simulink model "ssc_aircraft_ecs_data"  (Simulink 9.1)
settings: Solver=VariableStepAuto  StartTime=0.0  StopTime=6000  RelTol=1e-3  AbsTol=1e-3
PreLoadFcn:
  | p_init = 101.325; % kPa
  | T_init = 45; % degC
  | RH_init = 0.5;
  | O3_init = 0.05e-6;
  | 
  | R_O3 = 173.218; % J/(kg*K)
  | 
  | flow_area = 0.016; % m^2
  | 
  | D_fuselage = 4; % m
  | L_fuselage = 35; % m
undefined symbols (not defined in the file or in its folder): sigbuilder_block
libraries: fl_lib x57, nesl_utility x24, simulink x6, HVAC_lib x4
(part 1 of 2)
Description:
  | Aircraft Environmental Control System
  | 
  | Copyright 2017-2018 The MathWorks, Inc.
CloseFcn:
  | try,close(h1_ssc_aircraft_ecs),end
  | clear h1_ssc_aircraft_ecs
  | try,close(h2_ssc_aircraft_ecs),end
  | clear h2_ssc_aircraft_ecs
  | try,close(h3_ssc_aircraft_ecs),end
  | clear h3_ssc_aircraft_ecs
  | try,close(h4_ssc_aircraft_ecs),end
  | clear h4_ssc_aircraft_ecs
  | 
  | clear tout simlog_ssc_aircraft_ecs
  | clear p_init T_init RH_init O3_init R_O3 flow_area D_fuselage L_fuselage
settings Model: Creator=MathWorks  LastModifiedBy=ZENLAB-328
settings SolverCC: MaxConsecutiveMinStep=2
settings DataIOCC: SaveFormat=Dataset
settings OptimizationCC: LifeSpan=auto
settings DebuggingCC: UnderspecifiedInitializationDetection=Simplified  MergeDetectMultiDrivingBlocksExec=error  SFUnexpectedBacktrackingDiag=error  SFNoUnconditionalDefaultTransitionDiag=error  SFExecutionAtInitializationDiag=warning
settings HardwareCC: ProdBitPerPointer=64  ProdBitPerSizeT=64  ProdBitPerPtrDiffT=64  ProdLargestAtomicFloat=Float  ProdIntDivRoundTo=Zero  ProdEndianess=LittleEndian  ProdWordSize=64  ProdHWDeviceType=Intel->x86-64 (Windows64)
settings ModelReferenceCC: PropagateSignalLabelsOutOfModel=on
settings CodeAppCC: StateflowObjectComments=off
settings GRTTargetCC: TargetLangStandard=C99 (ISO)  CombineOutputUpdateFcns=on  GRTInterface=off
settings ConfigComp: CovMetricSettings=dwe  CovHtmlReporting=off  CovSaveCumulativeToWorkspaceVar=off  CovSaveSingleToWorkspaceVar=off  CovExternalEMLEnable=on
settings SimscapeCC: SimscapeLogType=all  SimscapeLogSimulationStatistics=on  SimscapeLogName=simlog_ssc_aircraft_ecs  SimscapeLogDataHistory=10000

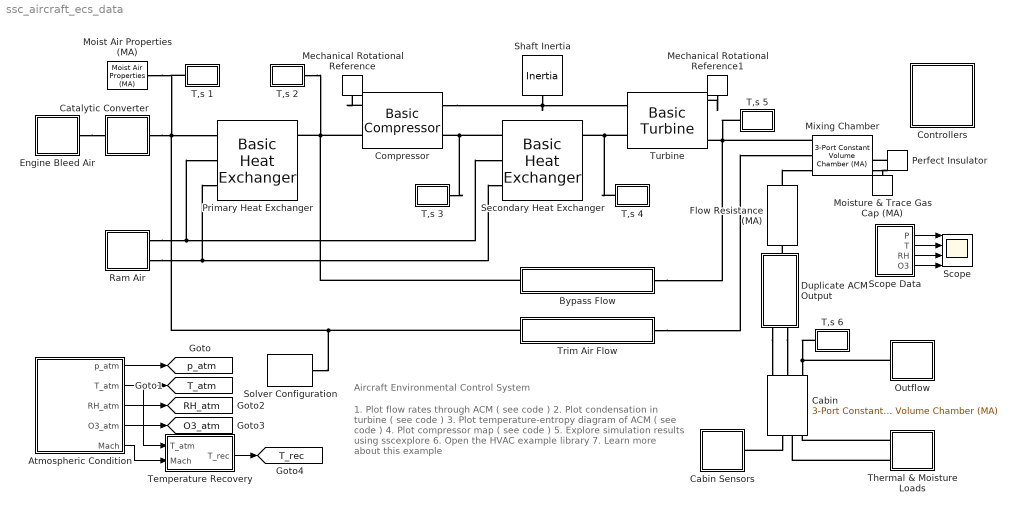
== system ssc_aircraft_ecs_data ==
  note: Aircraft Environmental Control System
  note: 1. Plot flow rates through ACM ( see code )
      | 2. Plot condensation in turbine ( see code )
      | 3. Plot temperature-entropy diagram of ACM ( see code )
      | 4. Plot compressor map ( see code )
      | 5. Explore simulation results using sscexplore
      | 6. Open the HVAC example library
      | 7. Learn more about this example
  Atmospheric Condition : Subsystem  Tag=STV Subsys  LoadFcn=sigbuilder_block('load');  StartFcn=sigbuilder_block('start');  StopFcn=sigbuilder_block('stop');  ClipboardFcn=sigbuilder_block('clipboard');  mask(Sigbuilder block){tuvar=[0:10]}
      mask help: Simulink:masks:SigbuilderBlock_MD
      mask init:
      | if ~strcmp(get_param(bdroot(gcbh),'SimulationStatus'),'stopped') tuvar = sigbuilder_block('maskInit'); end
      settings: CopyFcn=sigbuilder_block('copy');  DeleteFcn=sigbuilder_block('delete');  ModelCloseFcn=sigbuilder_block('modelClose');  PreSaveFcn=sigbuilder_block('preSave');  PauseFcn=sigbuilder_block('pause');  ContinueFcn=sigbuilder_block('continue');  NameChangeFcn=sigbuilder_block('namechange');  OpenFcn=sigbuilder_block('open',[42.75 9 1391.25 641.25 ]);  CloseFcn=sigbuilder_block('close');
      mask Display: plot(0, 0, 100, 100,[2, 2, 32, 32, 2], [68, 8, 8, 68, 68],[32, 2], [38, 38], [32, 19, 2],[53, 60, 44], [32, 17, 17, 2],[16, 16, 31, 31]);txt = getActiveGroup(gcbh);text(2, 100, txt,'verticalAlignment', 'top');
  Bypass Flow : Subsystem  Tag=PublishSubsystem
  Cabin : fl_lib/Moist Air/Elements/3-Port Constant Volume Chamber (MA)  volume=pi*D_fuselage^2/4 * L_fuselage m^3  area_A=flow_area m^2  area_B=flow_area m^2  area_C=flow_area m^2  RH_ws=1  time_constant=1e-3 s  p_I_specify=on  p_I_priority=High  p_I=p_init kPa  p_I_nominal_specify=off  p_I_nominal_unit=MPa  p_I_nominal_value=1  T_I_specify=on  T_I_priority=High  T_I=T_init degC  T_I_nominal_specify=off  T_I_nominal_unit=K  T_I_nominal_value=1  RH_I_specify=on  RH_I_priority=High  RH_I=RH_init  RH_I_nominal_specify=off  RH_I_nominal_unit=1  RH_I_nominal_value=1  x_w_I_specify=off  x_w_I_priority=None  x_w_I=0  x_w_I_nominal_specify=off  x_w_I_nominal_unit=1  x_w_I_nominal_value=1  y_w_I_specify=off  y_w_I_priority=None  y_w_I=0  y_w_I_nominal_specify=off  y_w_I_nominal_unit=1  y_w_I_nominal_value=1  HR_I_specify=off  HR_I_priority=None  HR_I=0  HR_I_nominal_specify=off  HR_I_nominal_unit=1  HR_I_nominal_value=1  x_g_I_specify=on  x_g_I_priority=None  x_g_I=0  x_g_I_nominal_specify=off  x_g_I_nominal_unit=1  x_g_I_nominal_value=1  y_g_I_specify=on  y_g_I_priority=High  y_g_I=O3_init  y_g_I_nominal_specify=off  y_g_I_nominal_unit=1  y_g_I_nominal_value=1  t_specify=off  t_priority=High  t=0 s  t_nominal_specify=off  t_nominal_unit=s  t_nominal_value=1
      settings: SourceProductName=Simscape  SourceProductBaseCode=SS
  Cabin Sensors : Subsystem
  Catalytic Converter : Subsystem  Tag=PublishSubsystem  mask(Catalytic Converter){}
      mask help: This subsystem removes ozone (O3) from the air flow at the specified removal rate.
      mask init:
      | removal_rate=evalin('base','Foz')
  Compressor : HVAC_lib/Basic Compressor  pr_des=2  mdot_corr_des=0.5 kg/s  omega_corr_des=4e4 rpm  p_ref=0.101325 MPa  T_ref=288.15 K  RH_ref=0  b1=1.5  b2=0.7  b3=0.08  eta_poly=0.92  eta_mech=0.98  area_A=flow_area m^2  area_B=flow_area/2 m^2  mdot_A_specify=off  mdot_A_priority=None  mdot_A=0 kg/s  mdot_A_nominal_specify=off  mdot_A_nominal_unit=kg/s  mdot_A_nominal_value=1  mdot_B_specify=off  mdot_B_priority=None  mdot_B=0 kg/s  mdot_B_nominal_specify=off  mdot_B_nominal_unit=kg/s  mdot_B_nominal_value=1  Phi_A_specify=off  Phi_A_priority=None  Phi_A=0 kW  Phi_A_nominal_specify=off  Phi_A_nominal_unit=kW  Phi_A_nominal_value=1  Phi_B_specify=off  Phi_B_priority=None  Phi_B=0 kW  Phi_B_nominal_specify=off  Phi_B_nominal_unit=kW  Phi_B_nominal_value=1  mdot_w_A_specify=off  mdot_w_A_priority=None  mdot_w_A=0 kg/s  mdot_w_A_nominal_specify=off  mdot_w_A_nominal_unit=kg/s  mdot_w_A_nominal_value=1  mdot_w_B_specify=off  mdot_w_B_priority=None  mdot_w_B=0 kg/s  mdot_w_B_nominal_specify=off  mdot_w_B_nominal_unit=kg/s  mdot_w_B_nominal_value=1  mdot_g_A_specify=off  mdot_g_A_priority=None  mdot_g_A=0 kg/s  mdot_g_A_nominal_specify=off  mdot_g_A_nominal_unit=kg/s  mdot_g_A_nominal_value=1  mdot_g_B_specify=off  mdot_g_B_priority=None  mdot_g_B=0 kg/s  mdot_g_B_nominal_specify=off  mdot_g_B_nominal_unit=kg/s  mdot_g_B_nominal_value=1  torque_specify=off  torque_priority=None  torque=1 N*m  torque_nominal_specify=off  torque_nominal_unit=N*m  torque_nominal_value=1  mechanical_power_specify=off  mechanical_power_priority=None  mechanical_power=1 kW  mechanical_power_nominal_specify=off  mechanical_power_nominal_unit=kW  mechanical_power_nominal_value=1  fluid_power_specify=off  fluid_power_priority=None  fluid_power=1 kW  fluid_power_nominal_specify=off  fluid_power_nominal_unit=kW  fluid_power_nominal_value=1  T_in_specify=off  T_in_priority=None  T_in=300 K  T_in_nominal_specify=off  T_in_nominal_unit=K  T_in_nominal_value=1  T_out_specify=off  T_out_priority=None  T_out=300 K  T_out_nominal_specify=off  T_out_nominal_unit=K  T_out_nominal_value=1
  Controllers : Subsystem  Tag=PublishSubsystem  mask(Controllers){T_turbine_setpoint=0, T_cabin_setpoint=22, p_cabin_min=80}
      mask prompts: T_turbine_setpoint "Turbine outlet temperature (degC)"; T_cabin_setpoint "Cabin temperature (degC)"; p_cabin_min "Minimum cabin pressure (kPa)"
      mask help: This subsystem contains the 4 controllers that regulate the flow in the air cycle machine (ACM) to achieve the following desired conditions.
      mask init:
      | mdot_setpoint=evalin('base','flowrate')
  Duplicate ACM Output : Subsystem  mask(Duplicate ACM Output){}
      mask help: This subsystem provides a second stream of conditioned air flow that mirrors the output of the first air cycle machine (ACM) without actually modeling the second ACM.
  Engine Bleed Air : Subsystem  Tag=PublishSubsystem  mask(Engine Bleed Air){p_bleed=250, T_bleed=180}
      mask prompts: p_bleed "Bleed air pressure (kPa)"; T_bleed "Bleed air temperature (degC)"
      mask help: This subsystem models the supply of hot, pressurized air to the air cycle machine (ACM) at a controlled flow rate.
  Flow Resistance (MA) : fl_lib/Moist Air/Elements/Flow Resistance (MA)  delta_p_nominal=1 kPa  mdot_nominal=1 kg/s  rho_nominal=1.2 kg/m^3  area=flow_area m^2  laminar_fraction=1e-3
      settings: SourceProductName=Simscape  SourceProductBaseCode=SS
  Mechanical Rotational Reference : fl_lib/Mechanical/Rotational Elements/Mechanical Rotational Reference
  Mechanical Rotational Reference1 : fl_lib/Mechanical/Rotational Elements/Mechanical Rotational Reference
  Mixing Chamber : fl_lib/Moist Air/Elements/3-Port Constant Volume Chamber (MA)  volume=0.001 m^3  area_A=flow_area m^2  area_B=flow_area m^2  area_C=flow_area m^2  RH_ws=1  time_constant=1e-3 s  p_I_specify=on  p_I_priority=High  p_I=p_init kPa  p_I_nominal_specify=off  p_I_nominal_unit=MPa  p_I_nominal_value=1  T_I_specify=on  T_I_priority=High  T_I=T_init degC  T_I_nominal_specify=off  T_I_nominal_unit=K  T_I_nominal_value=1  RH_I_specify=on  RH_I_priority=High  RH_I=RH_init  RH_I_nominal_specify=off  RH_I_nominal_unit=1  RH_I_nominal_value=1  x_w_I_specify=off  x_w_I_priority=None  x_w_I=0  x_w_I_nominal_specify=off  x_w_I_nominal_unit=1  x_w_I_nominal_value=1  y_w_I_specify=off  y_w_I_priority=None  y_w_I=0  y_w_I_nominal_specify=off  y_w_I_nominal_unit=1  y_w_I_nominal_value=1  HR_I_specify=off  HR_I_priority=None  HR_I=0  HR_I_nominal_specify=off  HR_I_nominal_unit=1  HR_I_nominal_value=1  x_g_I_specify=on  x_g_I_priority=None  x_g_I=0  x_g_I_nominal_specify=off  x_g_I_nominal_unit=1  x_g_I_nominal_value=1  y_g_I_specify=on  y_g_I_priority=High  y_g_I=O3_init  y_g_I_nominal_specify=off  y_g_I_nominal_unit=1  y_g_I_nominal_value=1  t_specify=off  t_priority=High  t=0 s  t_nominal_specify=off  t_nominal_unit=s  t_nominal_value=1
      settings: SourceProductName=Simscape  SourceProductBaseCode=SS
  Moist Air Properties (MA) : fl_lib/Moist Air/Utilities/Moist Air Properties (MA)  trace_gas_model=2  R_a=287.047 J/kg/K  R_w=461.523 J/kg/K  R_g=R_O3 J/kg/K  T_TLU=[-56.55, -50 : 10 : -10, -5 : 1 : 5, 10 : 10 : 350]' degC  p_ws_TLU=[1.71168953425982e-06; 3.93770601979424e-06; 1.28411717710344e-05; 3.80051394873809e-05; .00010323902900209; .000259873810798063; .000401741022116384; .000437454836117844; .000476040820618202; .000517704666185737; .000562664883741207; .000611212677444345; .000657088049117899; .000705987905898279; .000758082381149132; .000813549384183233; .000872574861129522; .00122818386934022; .0023392147667769; .00424668834054807; .00738442748706953; .0123512704340234; .0199458019246787; .0312006356960619; .0474147199263783; .0701823607447713; .10141797792131; .143375967241115; .198665399739302; .270259606559999; .361500961984849; .476101381081492; .618139196722055; .792053183687694; 1.0026345688121; 1.25501792086105; 1.55467186826983; 1.90739066433297; 2.31928772772542; 2.79679245576864; 3.34665187151016; 3.97593907083533; 4.69207105435535; 5.5028394740883; 6.41645928168037; 7.4416425436169; 8.58770832955728; 9.86474556030261; 11.2838558865497; 12.8575218898034; 14.6001810568052; 16.5291642526045] MPa  h_w_vap_TLU=[2836.88241275372; 2837.81392500514; 2838.63937175807; 2838.7309929628; 2838.06905313927; 2836.62597341095; 2835.60023952573; 2835.37006381376; 2835.13143158077; 2834.88429145066; 2834.62859062897; 2500.93420564316; 2498.55329907119; 2496.17495082036; 2493.79885912205; 2491.42474723191; 2489.05236104642; 2477.20875029194; 2453.54955988604; 2429.83856603313; 2406.00136954922; 2381.97406342174; 2357.69101156389; 2333.08088387814; 2308.06565480412; 2282.56034405021; 2256.47287422313; 2229.70428017508; 2202.14968030993; 2173.69998896199; 2144.24368406447; 2113.66758247452; 2081.85585110571; 2048.68725710494; 2014.03141249899; 1977.7449923284; 1939.66849592886; 1899.62342931686; 1857.40930169838; 1812.79975416601; 1765.53721731251; 1715.32525772152; 1661.81700477787; 1604.59703745016; 1543.1534616334; 1476.83692476464; 1404.80240352424; 1325.92091736114; 1238.61667822208; 1140.5102987018; 1027.62017777647; 892.733785613825] kJ/kg  h_a_TLU=[342.416126230579; 349.005511058471; 359.063577249119; 369.119948684177; 379.175469465129; 389.230944678417; 394.258910928084; 395.264534937366; 396.27017101329; 397.275819932805; 398.281482472874; 399.287159410541; 400.292851523015; 401.298559587728; 402.304284382408; 403.310026685143; 404.315787274435; 409.34489180313; 419.404921755863; 429.468036401264; 439.535033154839; 449.606720928652; 459.683919949603; 469.767460521911; 479.858181001348; 489.956925196484; 500.064539372946; 510.181869006204; 520.309755403634; 530.449032296018; 540.60052248087; 550.765034584465; 560.943359995745; 571.136270013102; 581.344513234296; 591.568813210327; 601.809866375885; 612.068340261954; 622.344871990218; 632.640067043998; 642.95449830646; 653.288705353699; 663.643193987949; 674.018435994423; 684.414869104228; 694.832897145098; 705.272890361557; 715.735185886199; 726.220088344236; 736.727870574087; 747.258774447567; 757.813011774199] kJ/kg  h_w_TLU=[2396.55944251649; 2408.68643343608; 2427.1988031141; 2445.702165897; 2464.18429108356; 2482.62529466839; 2491.82135326629; 2493.6580151792; 2495.49372578218; 2497.32843835745; 2499.16210446923; 2500.99462758899; 2502.83092214066; 2504.6665223621; 2506.50140563013; 2508.335548891; 2510.16892865793; 2519.32352241995; 2537.56068088674; 2555.67742615292; 2573.6403223998; 2591.4109179101; 2608.9455037701; 2626.19492016262; 2643.10444358428; 2659.61377634497; 2675.58278696023; 2696.1846256545; 2716.49989553741; 2736.6235210957; 2756.61216047011; 2776.50561773853; 2796.33378922508; 2816.11979583049; 2835.88181423877; 2855.63430574511; 2875.38889327595; 2895.15500577172; 2914.94035964689; 2934.75132290228; 2954.59319330244; 2974.47041285505; 2994.38673458964; 3014.34535328009; 3034.34900867103; 3054.40006755764; 3074.50058946898; 3094.65237953784; 3114.85703128106; 3135.11596137801; 3155.43043805905; 3175.80160435813] kJ/kg  h_g_TLU=-1 kJ/kg  mu_a_TLU=[14.2568883320012; 14.6140127728333; 15.1517277055779; 15.6806860159119; 16.2012351072083; 16.7137043125028; 16.9670071730589; 17.017438062815; 17.0677930842452; 17.1180725309876; 17.1682766951315; 17.2184058672268; 17.2684603362935; 17.3184403898301; 17.3683463138234; 17.4181783927569; 17.4679369096204; 17.7156358640698; 18.2056751785154; 18.68879035749; 19.1652344664982; 19.6352478927873; 20.099059103658; 20.5568853601578; 21.0089333871663; 21.4554000014051; 21.8964726992323; 22.3323302062775; 22.7631429910631; 23.1890737447833; 23.6102778293792; 24.0269036959922; 24.4390932757886; 24.8469823450548; 25.2507008663546; 25.6503733074314; 26.0461189394339; 26.4380521159325; 26.8262825340948; 27.2109154792923; 27.5920520543128; 27.969789394274; 28.3442208682439; 28.7154362685068; 29.0835219883356; 29.4485611890712; 29.8106339572472; 30.1698174524429; 30.5261860464955; 30.8798114546565; 31.2307628592324; 31.5791070262086] s*uPa  mu_w_TLU=[6.81365662228272; 7.04953750742707; 7.40970098298307; 7.76991278093907; 8.13017290129507; 8.49048134405107; 8.67065368632907; 8.70668960445667; 8.74272600580827; 8.77876289038387; 8.81480025818347; 8.85083810920707; 8.88687644345467; 8.92291526092627; 8.95895456162187; 8.99499434554147; 9.03103461268507; 9.21124319676307; 9.57169660671907; 9.93219833907507; 10.2927483938311; 10.6533467709871; 11.0139934705431; 11.3746884924991; 11.7354318368551; 12.0962235036111; 12.4570634927671; 12.8179518043231; 13.1788884382791; 13.5398733946351; 13.9009066733911; 14.2619882745471; 14.6231181981031; 14.9842964440591; 15.3455230124151; 15.7067979031711; 16.0681211163271; 16.4294926518831; 16.7909125098391; 17.1523806901951; 17.5138971929511; 17.8754620181071; 18.2370751656631; 18.5987366356191; 18.9604464279751; 19.3222045427311; 19.6840109798871; 20.0458657394431; 20.4077688213991; 20.7697202257551; 21.1317199525111; 21.4937680016671] s*uPa  mu_g_TLU=-1 s*uPa  k_a_TLU=[19.8808489374933; 20.4162454629695; 21.2248743590758; 22.0232452890903; 22.8117314495857; 23.5906913619588; 23.9767075412237; 24.053639990175; 24.1304826682191; 24.2072359051629; 24.2839000294007; 24.3604753679152; 24.4369622462801; 24.5133609886625; 24.5896719178249; 24.6658953551279; 24.7420316205333; 25.1214164701832; 25.8738283029331; 26.6180150229276; 27.3542674377332; 28.0828634735341; 28.8040686837224; 29.5181367785657; 30.2253101618423; 30.9258204644224; 31.6198890677835; 32.3077276126633; 32.9895384896798; 33.6655153099498; 34.33584335461; 35.0007000027879; 35.6602551380254; 36.3146715334901; 36.9641052165342; 37.6087058133173; 38.248616874307; 38.8839761815308; 39.5149160384798; 40.1415635435708; 40.7640408480637; 41.3824653993118; 41.9969501701893; 42.6076038755117; 43.2145311762238; 43.8178328720941; 44.4176060836121; 45.013944423749; 45.6069381602018; 46.1966743687041; 46.783237077953; 47.3667074066625] mW/m/K  k_w_TLU=[11.46288215976; 11.941997488935; 12.676358586935; 13.414208884935; 14.155548382935; 14.900377080935; 15.274099879935; 15.348949115735; 15.423833243535; 15.498752263335; 15.573706175135; 15.648694978935; 15.723718674735; 15.798777262535; 15.873870742335; 15.948999114135; 16.024162377935; 16.400502076935; 17.155798374935; 17.914583872935; 18.676858570935; 19.442622468935; 20.211875566935; 20.984617864935; 21.760849362935; 22.540570060935; 23.323779958935; 24.110479056935; 24.900667354935; 25.694344852935; 26.491511550935; 27.292167448935; 28.096312546935; 28.903946844935; 29.715070342935; 30.529683040935; 31.347784938935; 32.169376036935; 32.994456334935; 33.823025832935; 34.655084530935; 35.490632428935; 36.329669526935; 37.172195824935; 38.018211322935; 38.867716020935; 39.720709918935; 40.577193016935; 41.437165314935; 42.300626812935; 43.167577510935; 44.038017408935] mW/m/K  k_g_TLU=-1 mW/m/K  D_w=25 mm^2/s  D_g=16 mm^2/s  p_min=1 kPa  p_max=inf MPa  T_min=-56.55 degC  T_max=350 degC  p_atm=0.101325 MPa  T_atm=20 degC
      settings: SourceProductName=Simscape  SourceProductBaseCode=SS
  Moisture & Trace Gas Cap (MA) : fl_lib/Moist Air/Sources/Moisture & Trace Gas Sources/Moisture & Trace Gas Cap (MA)
      settings: SourceProductName=Simscape  SourceProductBaseCode=SS
  Outflow : Subsystem  Tag=PublishSubsystem
  Perfect Insulator : fl_lib/Thermal/Thermal Elements/Perfect Insulator  T_specify=off  T_priority=None  T=0 K  T_nominal_specify=off  T_nominal_unit=K  T_nominal_value=1
      settings: SourceProductName=Simscape
  Primary Heat Exchanger : HVAC_lib/Basic Heat Exchanger  Q_des=100 kW  T1_des=180 degC  mdot1_des=1 kg/s  cp1_des=1.02 kJ/kg/K  Dp1_des=20 kPa  T2_des=45 degC  mdot2_des=3 kg/s  cp2_des=1.007 kJ/kg/K  volume=0.025 m^3  port_area=flow_area m^2  RH_ws=1  time_constant=1e-3 s  p_I_specify=on  p_I_priority=High  p_I=p_init kPa  p_I_nominal_specify=off  p_I_nominal_unit=MPa  p_I_nominal_value=1  T_I_specify=on  T_I_priority=High  T_I=T_init degC  T_I_nominal_specify=off  T_I_nominal_unit=K  T_I_nominal_value=1  RH_I_specify=on  RH_I_priority=High  RH_I=RH_init  RH_I_nominal_specify=off  RH_I_nominal_unit=1  RH_I_nominal_value=1  x_w_I_specify=off  x_w_I_priority=None  x_w_I=0  x_w_I_nominal_specify=off  x_w_I_nominal_unit=1  x_w_I_nominal_value=1  y_w_I_specify=off  y_w_I_priority=None  y_w_I=0  y_w_I_nominal_specify=off  y_w_I_nominal_unit=1  y_w_I_nominal_value=1  HR_I_specify=off  HR_I_priority=None  HR_I=0  HR_I_nominal_specify=off  HR_I_nominal_unit=1  HR_I_nominal_value=1  x_g_I_specify=on  x_g_I_priority=None  x_g_I=0  x_g_I_nominal_specify=off  x_g_I_nominal_unit=1  x_g_I_nominal_value=1  y_g_I_specify=on  y_g_I_priority=High  y_g_I=O3_init  y_g_I_nominal_specify=off  y_g_I_nominal_unit=1  y_g_I_nominal_value=1  mdot_A_specify=off  mdot_A_priority=None  mdot_A=0 kg/s  mdot_A_nominal_specify=off  mdot_A_nominal_unit=kg/s  mdot_A_nominal_value=1  mdot_B_specify=off  mdot_B_priority=None  mdot_B=0 kg/s  mdot_B_nominal_specify=off  mdot_B_nominal_unit=kg/s  mdot_B_nominal_value=1  Phi_A_specify=off  Phi_A_priority=None  Phi_A=0 kW  Phi_A_nominal_specify=off  Phi_A_nominal_unit=kW  Phi_A_nominal_value=1  Phi_B_specify=off  Phi_B_priority=None  Phi_B=0 kW  Phi_B_nominal_specify=off  Phi_B_nominal_unit=kW  Phi_B_nominal_value=1  mdot_w_A_specify=off  mdot_w_A_priority=None  mdot_w_A=0 kg/s  mdot_w_A_nominal_specify=off  mdot_w_A_nominal_unit=kg/s  mdot_w_A_nominal_value=1  mdot_w_B_specify=off  mdot_w_B_priority=None  mdot_w_B=0 kg/s  mdot_w_B_nominal_specify=off  mdot_w_B_nominal_unit=kg/s  mdot_w_B_nominal_value=1  mdot_g_A_specify=off  mdot_g_A_priority=None  mdot_g_A=0 kg/s  mdot_g_A_nominal_specify=off  mdot_g_A_nominal_unit=kg/s  mdot_g_A_nominal_value=1  mdot_g_B_specify=off  mdot_g_B_priority=None  mdot_g_B=0 kg/s  mdot_g_B_nominal_specify=off  mdot_g_B_nominal_unit=kg/s  mdot_g_B_nominal_value=1  rho_I_specify=off  rho_I_priority=None  rho_I=1.2 kg/m^3  rho_I_nominal_specify=off  rho_I_nominal_unit=kg/m^3  rho_I_nominal_value=1  h_I_specify=off  h_I_priority=None  h_I=420 kJ/kg  h_I_nominal_specify=off  h_I_nominal_unit=kJ/kg  h_I_nominal_value=1  x_a_I_specify=off  x_a_I_priority=None  x_a_I=1  x_a_I_nominal_specify=off  x_a_I_nominal_unit=1  x_a_I_nominal_value=1  effectiveness_specify=off  effectiveness_priority=None  effectiveness=1  effectiveness_nominal_specify=off  effectiveness_nominal_unit=1  effectiveness_nominal_value=1  Q_hex_specify=off  Q_hex_priority=None  Q_hex=0 kW  Q_hex_nominal_specify=off  Q_hex_nominal_unit=kW  Q_hex_nominal_value=1  p_ws_ratio_I_specify=off  p_ws_ratio_I_priority=None  p_ws_ratio_I=1  p_ws_ratio_I_nominal_specify=off  p_ws_ratio_I_nominal_unit=1  p_ws_ratio_I_nominal_value=1  t_specify=off  t_priority=High  t=0 s  t_nominal_specify=off  t_nominal_unit=s  t_nominal_value=1
  Ram Air : Subsystem  mask(Ram Air){mdot_ram=3}
      mask prompts: mdot_ram "Ram air mass flow rate (kg/s)"
      mask help: This subsystem represents the air from the external environment that is used as the coolant for the heat exchangers in the air cycle machine (ACM).
  Scope : Scope  NumInputPorts=4
  Scope Data : Subsystem
      mask init:
      | %set_param([gcb,'/To Workspace'], 'VariableName', p_atm);
      | %set_param([gcb,'/To Workspace'], 'VariableName', p_cabin);
      | %set_param([gcb,'/To Workspace'], 'VariableName', T_cabin);
      | %set_param([gcb,'/To Workspace'], 'VariableName', RH_cabin);
      | %set_param([gcb,'/To Workspace'], 'VariableName', Q3_cabin);
  Secondary Heat Exchanger : HVAC_lib/Basic Heat Exchanger  Q_des=150 kW  T1_des=180 degC  mdot1_des=1 kg/s  cp1_des=1.02 kJ/kg/K  Dp1_des=20 kPa  T2_des=45 degC  mdot2_des=3 kg/s  cp2_des=1.007 kJ/kg/K  volume=0.025 m^3  port_area=flow_area/2 m^2  RH_ws=1  time_constant=1e-3 s  p_I_specify=on  p_I_priority=High  p_I=p_init kPa  p_I_nominal_specify=off  p_I_nominal_unit=MPa  p_I_nominal_value=1  T_I_specify=on  T_I_priority=High  T_I=T_init degC  T_I_nominal_specify=off  T_I_nominal_unit=K  T_I_nominal_value=1  RH_I_specify=on  RH_I_priority=High  RH_I=RH_init  RH_I_nominal_specify=off  RH_I_nominal_unit=1  RH_I_nominal_value=1  x_w_I_specify=off  x_w_I_priority=None  x_w_I=0  x_w_I_nominal_specify=off  x_w_I_nominal_unit=1  x_w_I_nominal_value=1  y_w_I_specify=off  y_w_I_priority=None  y_w_I=0  y_w_I_nominal_specify=off  y_w_I_nominal_unit=1  y_w_I_nominal_value=1  HR_I_specify=off  HR_I_priority=None  HR_I=0  HR_I_nominal_specify=off  HR_I_nominal_unit=1  HR_I_nominal_value=1  x_g_I_specify=on  x_g_I_priority=None  x_g_I=0  x_g_I_nominal_specify=off  x_g_I_nominal_unit=1  x_g_I_nominal_value=1  y_g_I_specify=on  y_g_I_priority=High  y_g_I=O3_init  y_g_I_nominal_specify=off  y_g_I_nominal_unit=1  y_g_I_nominal_value=1  mdot_A_specify=off  mdot_A_priority=None  mdot_A=0 kg/s  mdot_A_nominal_specify=off  mdot_A_nominal_unit=kg/s  mdot_A_nominal_value=1  mdot_B_specify=off  mdot_B_priority=None  mdot_B=0 kg/s  mdot_B_nominal_specify=off  mdot_B_nominal_unit=kg/s  mdot_B_nominal_value=1  Phi_A_specify=off  Phi_A_priority=None  Phi_A=0 kW  Phi_A_nominal_specify=off  Phi_A_nominal_unit=kW  Phi_A_nominal_value=1  Phi_B_specify=off  Phi_B_priority=None  Phi_B=0 kW  Phi_B_nominal_specify=off  Phi_B_nominal_unit=kW  Phi_B_nominal_value=1  mdot_w_A_specify=off  mdot_w_A_priority=None  mdot_w_A=0 kg/s  mdot_w_A_nominal_specify=off  mdot_w_A_nominal_unit=kg/s  mdot_w_A_nominal_value=1  mdot_w_B_specify=off  mdot_w_B_priority=None  mdot_w_B=0 kg/s  mdot_w_B_nominal_specify=off  mdot_w_B_nominal_unit=kg/s  mdot_w_B_nominal_value=1  mdot_g_A_specify=off  mdot_g_A_priority=None  mdot_g_A=0 kg/s  mdot_g_A_nominal_specify=off  mdot_g_A_nominal_unit=kg/s  mdot_g_A_nominal_value=1  mdot_g_B_specify=off  mdot_g_B_priority=None  mdot_g_B=0 kg/s  mdot_g_B_nominal_specify=off  mdot_g_B_nominal_unit=kg/s  mdot_g_B_nominal_value=1  rho_I_specify=off  rho_I_priority=None  rho_I=1.2 kg/m^3  rho_I_nominal_specify=off  rho_I_nominal_unit=kg/m^3  rho_I_nominal_value=1  h_I_specify=off  h_I_priority=None  h_I=420 kJ/kg  h_I_nominal_specify=off  h_I_nominal_unit=kJ/kg  h_I_nominal_value=1  x_a_I_specify=off  x_a_I_priority=None  x_a_I=1  x_a_I_nominal_specify=off  x_a_I_nominal_unit=1  x_a_I_nominal_value=1  effectiveness_specify=off  effectiveness_priority=None  effectiveness=1  effectiveness_nominal_specify=off  effectiveness_nominal_unit=1  effectiveness_nominal_value=1  Q_hex_specify=off  Q_hex_priority=None  Q_hex=0 kW  Q_hex_nominal_specify=off  Q_hex_nominal_unit=kW  Q_hex_nominal_value=1  p_ws_ratio_I_specify=off  p_ws_ratio_I_priority=None  p_ws_ratio_I=1  p_ws_ratio_I_nominal_specify=off  p_ws_ratio_I_nominal_unit=1  p_ws_ratio_I_nominal_value=1  t_specify=off  t_priority=High  t=0 s  t_nominal_specify=off  t_nominal_unit=s  t_nominal_value=1
  Shaft Inertia : fl_lib/Mechanical/Rotational Elements/Inertia  inertia=0.005 kg*m^2  w_specify=off  w_priority=High  w=0 rad/s  w_nominal_specify=off  w_nominal_unit=rad/s  w_nominal_value=1  t_specify=off  t_priority=None  t=0 N*m  t_nominal_specify=off  t_nominal_unit=N*m  t_nominal_value=1
  Solver Configuration : nesl_utility/Solver Configuration  PhysicalDomain=network_engine_domain  SubClassName=solver  LeftPortType=input  RightPortType=generic  Tones=[]  Harmonics=[]  SimulateNoise=off  Profile=off  UseLocalSampling=off  EnableSwitchedLinearOptims=on  FrequencyDomain=off  UseCCode=off  RelTol=0.001  AbsTol=1e-06  MinStep=1e-09  ToWorkspace=off  RevertToSquareIcSolve=off  NumHomotopyIterations=100  PhasorMode=off  PhasorModeNumHarmonics=1  DoDC=off  ResidualTolerance=1e-9  UseLocalSolver=off  LocalSolverChoice=NE_TRAPEZOIDAL_ADVANCER  LocalSolverSampleTime=0.01  DoFixedCost=off  MaxNonlinIter=3  MaxModeIter=2  LinearAlgebra=Sparse  EquationFormulation=NE_TIME_EF  DelaysMemoryBudget=1024  AutomaticFiltering=on  FilteringTimeConstant=0.001
  T,s 1 : Subsystem
      mask Display: disp(get_param(gcb, 'Name'))
  T,s 2 : Subsystem
      mask Display: disp(get_param(gcb, 'Name'))
  T,s 3 : Subsystem
      mask Display: disp(get_param(gcb, 'Name'))
  T,s 4 : Subsystem
      mask Display: disp(get_param(gcb, 'Name'))
  T,s 5 : Subsystem
      mask Display: disp(get_param(gcb, 'Name'))
  T,s 6 : Subsystem
      mask Display: disp(get_param(gcb, 'Name'))
  Temperature Recovery : Subsystem
  Thermal & Moisture Loads : Subsystem  Tag=PublishSubsystem  mask(Thermal & Moisture Loads){Q_passenger=70, W_passenger=0.04, T_passenger=30, hc_fuselage=2.5}
      mask prompts: Q_passenger "Sensible heat gain per passenger (W)"; W_passenger "Moisture gain per passenger (g/s)"; T_passenger "Exhalation temperature (degC)"; hc_fuselage "Fuselage heat transfer coefficient (W/(m^2*K))"
      mask help: This subsystem adds sources of heat and moisture to the cabin air volume.
      mask init:
      | N_passenger=evalin('base','P')
      | Q_equipment=evalin('base','Teq')
  Trim Air Flow : Subsystem  Tag=PublishSubsystem
  Turbine : HVAC_lib/Basic Turbine  pr_des=0.2  mdot_corr_des=0.22 kg/s  p_ref=0.101325 MPa  T_ref=288.15 K  RH_ref=0  eta_poly=0.92  eta_mech=0.98  area_A=flow_area/2 m^2  area_B=flow_area m^2  RH_ws=1  mdot_A_specify=off  mdot_A_priority=None  mdot_A=0 kg/s  mdot_A_nominal_specify=off  mdot_A_nominal_unit=kg/s  mdot_A_nominal_value=1  mdot_B_specify=off  mdot_B_priority=None  mdot_B=0 kg/s  mdot_B_nominal_specify=off  mdot_B_nominal_unit=kg/s  mdot_B_nominal_value=1  Phi_A_specify=off  Phi_A_priority=None  Phi_A=0 kW  Phi_A_nominal_specify=off  Phi_A_nominal_unit=kW  Phi_A_nominal_value=1  Phi_B_specify=off  Phi_B_priority=None  Phi_B=0 kW  Phi_B_nominal_specify=off  Phi_B_nominal_unit=kW  Phi_B_nominal_value=1  mdot_w_A_specify=off  mdot_w_A_priority=None  mdot_w_A=0 kg/s  mdot_w_A_nominal_specify=off  mdot_w_A_nominal_unit=kg/s  mdot_w_A_nominal_value=1  mdot_w_B_specify=off  mdot_w_B_priority=None  mdot_w_B=0 kg/s  mdot_w_B_nominal_specify=off  mdot_w_B_nominal_unit=kg/s  mdot_w_B_nominal_value=1  mdot_g_A_specify=off  mdot_g_A_priority=None  mdot_g_A=0 kg/s  mdot_g_A_nominal_specify=off  mdot_g_A_nominal_unit=kg/s  mdot_g_A_nominal_value=1  mdot_g_B_specify=off  mdot_g_B_priority=None  mdot_g_B=0 kg/s  mdot_g_B_nominal_specify=off  mdot_g_B_nominal_unit=kg/s  mdot_g_B_nominal_value=1  torque_specify=off  torque_priority=None  torque=1 N*m  torque_nominal_specify=off  torque_nominal_unit=N*m  torque_nominal_value=1  mechanical_power_specify=off  mechanical_power_priority=None  mechanical_power=1 kW  mechanical_power_nominal_specify=off  mechanical_power_nominal_unit=kW  mechanical_power_nominal_value=1  fluid_power_specify=off  fluid_power_priority=None  fluid_power=1 kW  fluid_power_nominal_specify=off  fluid_power_nominal_unit=kW  fluid_power_nominal_value=1  T_in_specify=off  T_in_priority=None  T_in=300 K  T_in_nominal_specify=off  T_in_nominal_unit=K  T_in_nominal_value=1  T_work_specify=off  T_work_priority=None  T_work=300 K  T_work_nominal_specify=off  T_work_nominal_unit=K  T_work_nominal_value=1  T_out_specify=off  T_out_priority=None  T_out=300 K  T_out_nominal_specify=off  T_out_nominal_unit=K  T_out_nominal_value=1  p_ws_ratio_out_specify=off  p_ws_ratio_out_priority=None  p_ws_ratio_out=1  p_ws_ratio_out_nominal_specify=off  p_ws_ratio_out_nominal_unit=1  p_ws_ratio_out_nominal_value=1
  tag scope: O3_atm=global, RH_atm=global, T_atm=global, T_rec=global, p_atm=global
  wires:
  Atmospheric Condition/1(p_atm) -> [p_atm]
  Atmospheric Condition/2(T_atm) -> Temperature Recovery/1(T_atm), [T_atm]
  Atmospheric Condition/3(RH_atm) -> [RH_atm]
  Atmospheric Condition/5(Mach) -> Temperature Recovery/2(Mach)
  Atmospheric Condition/4(O3_atm) -> [O3_atm]
  Temperature Recovery/1(T_rec) -> [T_rec]
  Scope Data/1(P) -> Scope/1
  Scope Data/2(T) -> Scope/2
  Scope Data/3(RH) -> Scope/3
  Scope Data/4(O3) -> Scope/4
  connections:
  Compressor/LConn1 -- T,s 2/LConn1 -- Bypass Flow/LConn1 -- Primary Heat Exchanger/RConn1
  Secondary Heat Exchanger/LConn1 -- T,s 3/LConn1 -- Compressor/RConn1
  Turbine/LConn1 -- Secondary Heat Exchanger/RConn1 -- T,s 4/LConn1
  Compressor/RConn2 -- Shaft Inertia/LConn1 -- Turbine/LConn2
  Mechanical Rotational Reference1/LConn1 -- Turbine/RConn3
  Perfect Insulator/LConn1 -- Mixing Chamber/RConn3
  Bypass Flow/RConn1 -- T,s 5/LConn1 -- Mixing Chamber/LConn1 -- Turbine/RConn1
  Trim Air Flow/LConn1 -- Solver Configuration/RConn1 -- Moist Air Properties (MA)/RConn1 -- T,s 1/LConn1 -- Primary Heat Exchanger/LConn1 -- Catalytic Converter/RConn1
  Trim Air Flow/RConn1 -- Mixing Chamber/LConn2
  Flow Resistance (MA)/LConn1 -- Mixing Chamber/LConn3
  Compressor/LConn2 -- Mechanical Rotational Reference/LConn1
  Mixing Chamber/RConn4 -- Moisture & Trace Gas Cap (MA)/LConn1
  Duplicate ACM Output/LConn1 -- Flow Resistance (MA)/RConn1
  Duplicate ACM Output/RConn1 -- Cabin/LConn1
  Duplicate ACM Output/RConn2 -- Cabin/LConn2
  T,s 6/LConn1 -- Outflow/LConn1 -- Cabin/LConn3
  Thermal & Moisture Loads/RConn1 -- Cabin/RConn4
  Thermal & Moisture Loads/RConn2 -- Cabin/RConn3
  Cabin/RConn2 -- Cabin Sensors/RConn1
  Ram Air/RConn1 -- Secondary Heat Exchanger/LConn2 -- Primary Heat Exchanger/LConn2
  Ram Air/RConn2 -- Secondary Heat Exchanger/LConn3 -- Primary Heat Exchanger/LConn3
  Engine Bleed Air/RConn1 -- Catalytic Converter/LConn1

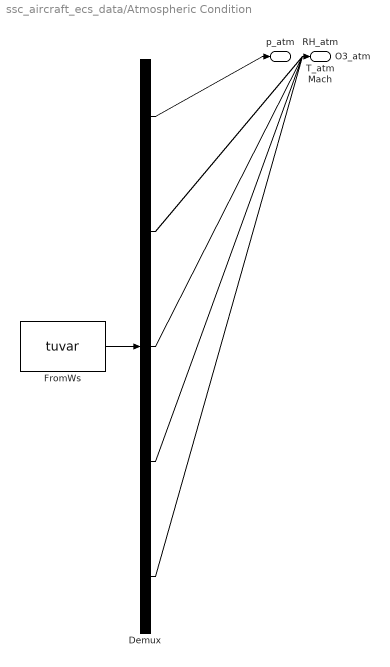
== system ssc_aircraft_ecs_data/Atmospheric Condition ==
  Demux : Demux  Tag=STV Demux  Outputs=5
  FromWs : FromWorkspace  Tag=STV FromWs  VariableName=tuvar  SampleTime=0  SigBuilderData=DataTag0  VnvData=DataTag1
      SigBuilderData=|
      | common.afterFinalStr = 'Extrapolate'
      | common.sampleTime = '0'
      | dataSet.timeRange = [0 6000]
      | dataSet.name = 'Group 1'
      | sbobj.Groups.Name = 'Group 1'
      | sbobj.Groups.Signals(1).Name = 'p_atm'
      | sbobj.Groups.Signals(1).XData = [0 600 1800 4200 5400 6000]
      | sbobj.Groups.Signals(1).YData = [101.325 101.325 22 22 101.325 101.325]
      | sbobj.Groups.Signals(2).Name = 'T_atm'
      | sbobj.Groups.Signals(2).XData = [0 600 1800 4200 5500 6000]
      | sbobj.Groups.Signals(2).YData = [45 45 -55 -55 -30 -30]
      | sbobj.Groups.Signals(3).Name = 'RH_atm'
      | sbobj.Groups.Signals(3).XData = [0 4200 5400 6000]
      | sbobj.Groups.Signals(3).YData = [0.5 0.5 0.9 0.9]
      | sbobj.Groups.Signals(4).Name = 'O3_atm'
      | sbobj.Groups.Signals(4).XData = [0 600 1100 1800 4200 5400 6000]
      | sbobj.Groups.Signals(4).YData = [0.05 0.05 0.024 0.09 0.09 0.02 0.02]
      | sbobj.Groups.Signals(5).Name = 'Mach'
      | sbobj.Groups.Signals(5).XData = [0 600 1800 4200 6000]
      | sbobj.Groups.Signals(5).YData = [0 0 0.8 0.8 0.773548387097]
      | sbobj.Groups.TimeRange = [0 6000]
  p_atm : Outport  Tag=STV Outport
  T_atm : Outport  Tag=STV Outport  Port=2
  RH_atm : Outport  Tag=STV Outport  Port=3
  O3_atm : Outport  Tag=STV Outport  Port=4
  Mach : Outport  Tag=STV Outport  Port=5
  wires:
  FromWs/1 -> Demux/1
  Demux/1 -> p_atm/1
  Demux/2 -> T_atm/1
  Demux/3 -> RH_atm/1
  Demux/4 -> O3_atm/1
  Demux/5 -> Mach/1

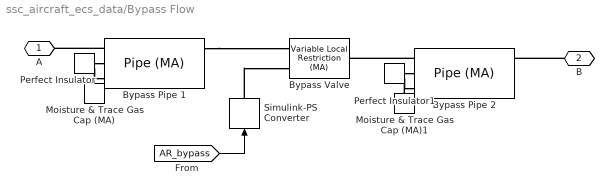
== system ssc_aircraft_ecs_data/Bypass Flow ==
  Bypass Pipe 1 : fl_lib/Moist Air/Elements/Pipe (MA)  length=0.5 m  area=flow_area m^2  Dh=sqrt(flow_area*4/pi) m  length_add=0.05 m  roughness=15e-6 m  Re_lam=2000  Re_tur=4000  shape_factor=64  Nu_lam=3.66  RH_ws=1  time_constant=1e-3 s  p_I_specify=on  p_I_priority=High  p_I=p_init kPa  p_I_nominal_specify=off  p_I_nominal_unit=MPa  p_I_nominal_value=1  T_I_specify=on  T_I_priority=High  T_I=T_init degC  T_I_nominal_specify=off  T_I_nominal_unit=K  T_I_nominal_value=1  RH_I_specify=on  RH_I_priority=High  RH_I=RH_init  RH_I_nominal_specify=off  RH_I_nominal_unit=1  RH_I_nominal_value=1  x_w_I_specify=off  x_w_I_priority=None  x_w_I=0  x_w_I_nominal_specify=off  x_w_I_nominal_unit=1  x_w_I_nominal_value=1  y_w_I_specify=off  y_w_I_priority=None  y_w_I=0  y_w_I_nominal_specify=off  y_w_I_nominal_unit=1  y_w_I_nominal_value=1  HR_I_specify=off  HR_I_priority=None  HR_I=0  HR_I_nominal_specify=off  HR_I_nominal_unit=1  HR_I_nominal_value=1  x_g_I_specify=on  x_g_I_priority=None  x_g_I=0  x_g_I_nominal_specify=off  x_g_I_nominal_unit=1  x_g_I_nominal_value=1  y_g_I_specify=on  y_g_I_priority=High  y_g_I=O3_init  y_g_I_nominal_specify=off  y_g_I_nominal_unit=1  y_g_I_nominal_value=1  t_specify=off  t_priority=High  t=0 s  t_nominal_specify=off  t_nominal_unit=s  t_nominal_value=1
      settings: SourceProductName=Simscape  SourceProductBaseCode=SS
  Bypass Pipe 2 : fl_lib/Moist Air/Elements/Pipe (MA)  length=0.5 m  area=flow_area m^2  Dh=sqrt(flow_area*4/pi) m  length_add=0.05 m  roughness=15e-6 m  Re_lam=2000  Re_tur=4000  shape_factor=64  Nu_lam=3.66  RH_ws=1  time_constant=1e-3 s  p_I_specify=on  p_I_priority=High  p_I=p_init kPa  p_I_nominal_specify=off  p_I_nominal_unit=MPa  p_I_nominal_value=1  T_I_specify=on  T_I_priority=High  T_I=T_init degC  T_I_nominal_specify=off  T_I_nominal_unit=K  T_I_nominal_value=1  RH_I_specify=on  RH_I_priority=High  RH_I=RH_init  RH_I_nominal_specify=off  RH_I_nominal_unit=1  RH_I_nominal_value=1  x_w_I_specify=off  x_w_I_priority=None  x_w_I=0  x_w_I_nominal_specify=off  x_w_I_nominal_unit=1  x_w_I_nominal_value=1  y_w_I_specify=off  y_w_I_priority=None  y_w_I=0  y_w_I_nominal_specify=off  y_w_I_nominal_unit=1  y_w_I_nominal_value=1  HR_I_specify=off  HR_I_priority=None  HR_I=0  HR_I_nominal_specify=off  HR_I_nominal_unit=1  HR_I_nominal_value=1  x_g_I_specify=on  x_g_I_priority=None  x_g_I=0  x_g_I_nominal_specify=off  x_g_I_nominal_unit=1  x_g_I_nominal_value=1  y_g_I_specify=on  y_g_I_priority=High  y_g_I=O3_init  y_g_I_nominal_specify=off  y_g_I_nominal_unit=1  y_g_I_nominal_value=1  t_specify=off  t_priority=High  t=0 s  t_nominal_specify=off  t_nominal_unit=s  t_nominal_value=1
      settings: SourceProductName=Simscape  SourceProductBaseCode=SS
  Bypass Valve : fl_lib/Moist Air/Elements/Variable Local Restriction (MA)  min_area=1e-10 m^2  max_area=0.98*flow_area m^2  area=flow_area m^2  Cd=0.8  B_lam=0.999
      settings: SourceProductName=Simscape  SourceProductBaseCode=SS
  Moisture & Trace Gas Cap (MA) : fl_lib/Moist Air/Sources/Moisture & Trace Gas Sources/Moisture & Trace Gas Cap (MA)
      settings: SourceProductName=Simscape  SourceProductBaseCode=SS
  Moisture & Trace Gas Cap (MA)1 : fl_lib/Moist Air/Sources/Moisture & Trace Gas Sources/Moisture & Trace Gas Cap (MA)
      settings: SourceProductName=Simscape  SourceProductBaseCode=SS
  Perfect Insulator : fl_lib/Thermal/Thermal Elements/Perfect Insulator  T_specify=off  T_priority=None  T=0 K  T_nominal_specify=off  T_nominal_unit=K  T_nominal_value=1
      settings: SourceProductName=Simscape
  Perfect Insulator1 : fl_lib/Thermal/Thermal Elements/Perfect Insulator  T_specify=off  T_priority=None  T=0 K  T_nominal_specify=off  T_nominal_unit=K  T_nominal_value=1
      settings: SourceProductName=Simscape
  Simulink-PS Converter : nesl_utility/Simulink-PS Converter  PhysicalDomain=network_engine_domain  SubClassName=ps_input  LeftPortType=input  RightPortType=output  PseudoPeriodic=off  Frequencies=[]  NoiseDistribution=none  NoiseParameters=[]  Unit=m^2  AffineConversion=off  FilteringAndDerivatives=provide  SimscapeFilterOrder=1  InputFilterTimeConstant=0.001  UdotUserProvided=0
  A : PMIOPort  Side=Left
  B : PMIOPort  Port=2  Side=Right
  wires:
  [AR_bypass] -> Simulink-PS Converter/1
  connections:
  Bypass Pipe 1/LConn1 -- A/RConn1
  Bypass Pipe 1/RConn1 -- Bypass Valve/LConn1
  Moisture & Trace Gas Cap (MA)/LConn1 -- Bypass Pipe 1/LConn3
  Perfect Insulator/LConn1 -- Bypass Pipe 1/LConn2
  Perfect Insulator1/LConn1 -- Bypass Pipe 2/LConn2
  Moisture & Trace Gas Cap (MA)1/LConn1 -- Bypass Pipe 2/LConn3
  Bypass Pipe 2/LConn1 -- Bypass Valve/RConn1
  B/RConn1 -- Bypass Pipe 2/RConn1
  Simulink-PS Converter/RConn1 -- Bypass Valve/LConn2

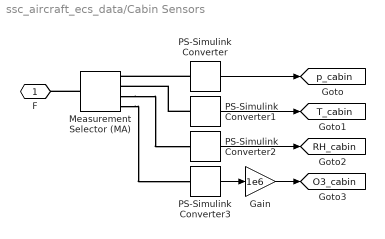
== system ssc_aircraft_ecs_data/Cabin Sensors ==
  Gain : Gain  Gain=1e6
  Measurement Selector (MA) : fl_lib/Moist Air/Sensors/Measurement Selector (MA)  moisture_spec=foundation.enum.moisture_spec.relative_humidity  trace_gas_spec=foundation.enum.trace_gas_spec.mole_fraction
      settings: SourceProductName=Simscape  SourceProductBaseCode=SS
  PS-Simulink Converter : nesl_utility/PS-Simulink Converter  PhysicalDomain=network_engine_domain  SubClassName=ps_output  LeftPortType=input  RightPortType=output  PseudoPeriodic=off  Frequencies=[]  Unit=kPa  AffineConversion=off
  PS-Simulink Converter1 : nesl_utility/PS-Simulink Converter  PhysicalDomain=network_engine_domain  SubClassName=ps_output  LeftPortType=input  RightPortType=output  PseudoPeriodic=off  Frequencies=[]  Unit=degC  AffineConversion=on
  PS-Simulink Converter2 : nesl_utility/PS-Simulink Converter  PhysicalDomain=network_engine_domain  SubClassName=ps_output  LeftPortType=input  RightPortType=output  PseudoPeriodic=off  Frequencies=[]  Unit=1  AffineConversion=off
  PS-Simulink Converter3 : nesl_utility/PS-Simulink Converter  PhysicalDomain=network_engine_domain  SubClassName=ps_output  LeftPortType=input  RightPortType=output  PseudoPeriodic=off  Frequencies=[]  Unit=1  AffineConversion=off
  F : PMIOPort  Side=Right
  tag scope: O3_cabin=global, RH_cabin=global, T_cabin=global, p_cabin=global
  wires:
  PS-Simulink Converter/1 -> [p_cabin]
  PS-Simulink Converter1/1 -> [T_cabin]
  PS-Simulink Converter2/1 -> [RH_cabin]
  PS-Simulink Converter3/1 -> Gain/1
  Gain/1 -> [O3_cabin]
  connections:
  Measurement Selector (MA)/LConn1 -- F/RConn1
  PS-Simulink Converter/LConn1 -- Measurement Selector (MA)/RConn1
  PS-Simulink Converter1/LConn1 -- Measurement Selector (MA)/RConn2
  Measurement Selector (MA)/RConn3 -- PS-Simulink Converter2/LConn1
  Measurement Selector (MA)/RConn4 -- PS-Simulink Converter3/LConn1

== system ssc_aircraft_ecs_data/Catalytic Converter ==
  Controlled Trace Gas Source (MA) : fl_lib/Moist Air/Sources/Moisture & Trace Gas Sources/Controlled Trace Gas Source (MA)
      settings: SourceProductName=Simscape  SourceProductBaseCode=SS
  Mass & Energy Flow Rate Sensor (MA) : fl_lib/Moist Air/Sensors/Mass & Energy Flow Rate Sensor (MA)
      settings: SourceProductName=Simscape  SourceProductBaseCode=SS
  Perfect Insulator : fl_lib/Thermal/Thermal Elements/Perfect Insulator  T_specify=off  T_priority=None  T=0 K  T_nominal_specify=off  T_nominal_unit=K  T_nominal_value=1
      settings: SourceProductName=Simscape
  Pipe (MA) : fl_lib/Moist Air/Elements/Pipe (MA)  length=0.5 m  area=flow_area m^2  Dh=sqrt(flow_area*4/pi) m  length_add=0.05 m  roughness=15e-6 m  Re_lam=2000  Re_tur=4000  shape_factor=64  Nu_lam=3.66  RH_ws=1  time_constant=1e-3 s  p_I_specify=on  p_I_priority=High  p_I=p_init kPa  p_I_nominal_specify=off  p_I_nominal_unit=MPa  p_I_nominal_value=1  T_I_specify=on  T_I_priority=High  T_I=T_init degC  T_I_nominal_specify=off  T_I_nominal_unit=K  T_I_nominal_value=1  RH_I_specify=on  RH_I_priority=High  RH_I=RH_init  RH_I_nominal_specify=off  RH_I_nominal_unit=1  RH_I_nominal_value=1  x_w_I_specify=off  x_w_I_priority=None  x_w_I=0  x_w_I_nominal_specify=off  x_w_I_nominal_unit=1  x_w_I_nominal_value=1  y_w_I_specify=off  y_w_I_priority=None  y_w_I=0  y_w_I_nominal_specify=off  y_w_I_nominal_unit=1  y_w_I_nominal_value=1  HR_I_specify=off  HR_I_priority=None  HR_I=0  HR_I_nominal_specify=off  HR_I_nominal_unit=1  HR_I_nominal_value=1  x_g_I_specify=on  x_g_I_priority=None  x_g_I=0  x_g_I_nominal_specify=off  x_g_I_nominal_unit=1  x_g_I_nominal_value=1  y_g_I_specify=on  y_g_I_priority=High  y_g_I=O3_init  y_g_I_nominal_specify=off  y_g_I_nominal_unit=1  y_g_I_nominal_value=1  t_specify=off  t_priority=High  t=0 s  t_nominal_specify=off  t_nominal_unit=s  t_nominal_value=1
      settings: SourceProductName=Simscape  SourceProductBaseCode=SS
  Removal Rate : fl_lib/Physical Signals/Functions/PS Gain  gain=-removal_rate
  A : PMIOPort  Side=Left
  B : PMIOPort  Port=2  Side=Right
  connections:
  Removal Rate/RConn1 -- Controlled Trace Gas Source (MA)/RConn1
  Mass & Energy Flow Rate Sensor (MA)/LConn1 -- A/RConn1
  Mass & Energy Flow Rate Sensor (MA)/LConn3 -- Removal Rate/LConn1
  Pipe (MA)/RConn1 -- B/RConn1
  Pipe (MA)/LConn2 -- Perfect Insulator/LConn1
  Pipe (MA)/LConn3 -- Controlled Trace Gas Source (MA)/LConn1
  Pipe (MA)/LConn1 -- Mass & Energy Flow Rate Sensor (MA)/RConn1
